simulink model "ss_lin"  (Simulink 2.20)
settings: Solver=FixedStepDiscrete  StartTime=0.0  StopTime=10.0  RelTol=1e-3  AbsTol=1e-6
values from neighbouring files (symbols this model uses):
  C = [-k3 0 -k2 0;1 0 0 0; 0 1 0 0;0 0 1 0;0 0 0 1]    [tilstandmodel_lang_pind.m]
  D = [0;0;0;0;0]    [tilstandmodel_lang_pind.m]
  K = acker(Phi, Gamma, pz)    [tilstandmodel_lang_pind.m]
  k2 = 1.43688    [tilstandmodel_lang_pind.m]
  k3 = 6.41894    [tilstandmodel_lang_pind.m]
  kr1 = Phi_r(2,1)-Lr*Phi_r(1,1)    [tilstandmodel_lang_pind.m]
  kr2 = Phi_r(2,2)-Lr*Phi_r(1,2)    [tilstandmodel_lang_pind.m]
  kr3 = Gamma_r(2)-Lr*Gamma_r(1)    [tilstandmodel_lang_pind.m]
  Lr = (Phi_r(2,2) -pze)/Phi_r(1,2)    [tilstandmodel_lang_pind.m]
  ref = 0    [tilstandmodel_lang_pind.m]
undefined symbols (not defined in the file or in its folder): Gamma, Phi
libraries: simulink x2
settings Model: ConsistencyChecking=off  RTWPlaceOutputsASAP=off

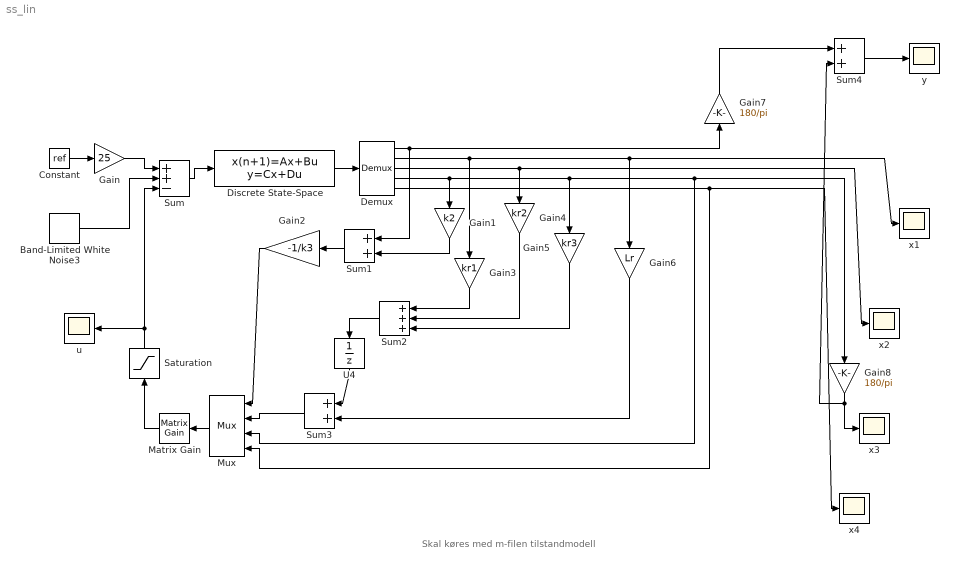
== system ss_lin ==
  note: Skal køres med m-filen tilstandmodell
  Band-Limited White Noise3 : simulink/Sources/Band-Limited White Noise  Cov=[0.2]  Ts=0.025  seed=[23341]
  Constant : Constant  Value=ref
  Demux : Demux  Outputs=5
  Discrete State-Space : DiscreteStateSpace  A=Phi  B=Gamma  C=C  D=D  X0=0  SampleTime=0.025
  Gain : Gain  Gain=25
  Gain1 : Gain  Orientation=down  Gain=k2
  Gain2 : Gain  Orientation=left  Gain=-1/k3
  Gain3 : Gain  Orientation=down  Gain=kr1
  Gain4 : Gain  Orientation=down  Gain=kr2
  Gain5 : Gain  Orientation=down  Gain=kr3
  Gain6 : Gain  Orientation=down  Gain=Lr
  Gain7 : Gain  Orientation=up  Gain=180/pi
  Gain8 : Gain  Orientation=down  Gain=180/pi
  Matrix Gain : simulink/Linear/Matrix Gain  Orientation=left  K=K
  Mux : Mux  Orientation=left  Inputs=4
  Saturation : Saturate  Orientation=up  UpperLimit=5  LowerLimit=-5
  Sum : Sum  Inputs=++-
  Sum1 : Sum  Orientation=left  Inputs=++
  Sum2 : Sum  Orientation=left  Inputs=+++
  Sum3 : Sum  Orientation=left  Inputs=++
  Sum4 : Sum  Inputs=++
  U4 : UnitDelay  Orientation=down  X0=0  SampleTime=0.025
  u : Scope
      settings: TickLabels=on  TimeRange=auto  YMin=-5  YMax=5  SaveToWorkspace=off  SaveName=ScopeData  LimitMaxRows=off
  x{1..4} (4 alike) : Scope
      settings: TickLabels=on  TimeRange=auto  YMin=-5  YMax=5  SaveToWorkspace=off  SaveName=ScopeData  LimitMaxRows=off
  y : Scope
      settings: TickLabels=on  TimeRange=auto  YMin=-5  YMax=5  SaveToWorkspace=off  SaveName=ScopeData  LimitMaxRows=off
  wires:
  Constant/1 -> Gain/1
  Gain/1 -> Sum/1
  Sum/1 -> Discrete State-Space/1
  Demux/1 -> Sum1/1, Gain7/1
  Demux/4 -> Gain1/1, Mux/3, Gain8/1, Gain5/1
  Gain1/1 -> Sum1/2
  Sum1/1 -> Gain2/1
  Mux/1 -> Matrix Gain/1
  Gain2/1 -> Mux/1
  Sum3/1 -> Mux/2
  Gain6/1 -> Sum3/2
  Sum2/1 -> U4/1
  U4/1 -> Sum3/1
  Gain3/1 -> Sum2/1
  Gain4/1 -> Sum2/2
  Gain5/1 -> Sum2/3
  Matrix Gain/1 -> Saturation/1
  Discrete State-Space/1 -> Demux/1
  Demux/5 -> x4/1, Mux/4
  Demux/3 -> Gain4/1, x2/1
  Gain7/1 -> Sum4/1
  Gain8/1 -> x3/1, Sum4/2
  Sum4/1 -> y/1
  Demux/2 -> Gain3/1, x1/1, Gain6/1
  Band-Limited White Noise3/1 -> Sum/2
  Saturation/1 -> u/1, Sum/3
